simulink model "Simulation"  (R2023a)
settings: Solver=VariableStepAuto  StartTime=0.0  StopTime=100.0  RelTol=1e-3
settings Model: Creator=thoma  LastModifiedBy=cheva

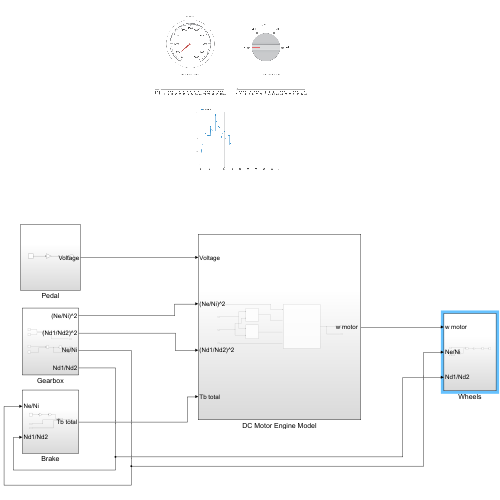
[thumbnail: Simulink's stored preview of the top-level diagram]
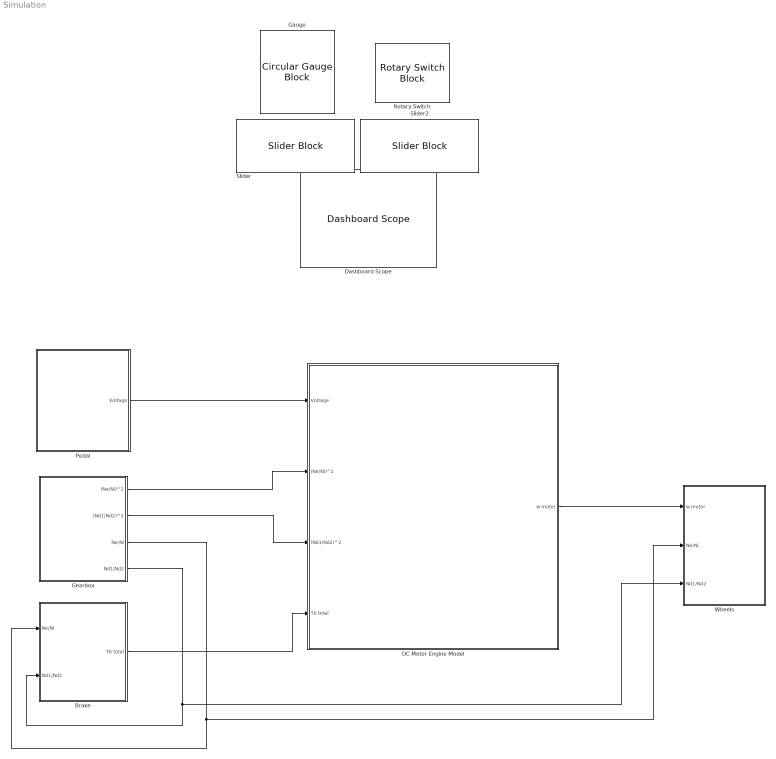
== system Simulation ==
  Brake : Subsystem
  DC Motor Engine Model : Subsystem
  Dashboard Scope : DashboardScope  Ymin=0  Ymax=10000
  Gauge : CircularGaugeBlock  ScaleMax=5000
  Gearbox : Subsystem
  Pedal : Subsystem
  Rotary Switch : RotarySwitchBlock
      settings: Values={{'1st', '2nd', '3rd', '4th'}, [3 2 1.5 1]}
  Slider : SliderBlock
  Slider2 : SliderBlock
  Wheels : Subsystem
  wires:
  Gearbox/4(Nd1/Nd2) -> Brake/2(Nd1/Nd2), Wheels/3(Nd1/Nd2)
  Gearbox/3(Ne/Ni) -> Brake/1(Ne/Ni), Wheels/2(Ne/Ni)
  Pedal/1(Voltage) -> DC Motor Engine Model/1(Voltage)
  Gearbox/1((Ne/Ni)^2) -> DC Motor Engine Model/2((Ne/Ni)^2)
  Gearbox/2((Nd1/Nd2)^2) -> DC Motor Engine Model/3((Nd1/Nd2)^2)
  Brake/1(Tb total) -> DC Motor Engine Model/4(Tb total)
  DC Motor Engine Model/1("w motor ") -> Wheels/1(w motor)

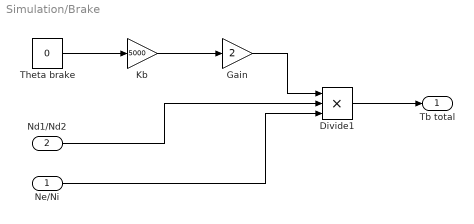
== system Simulation/Brake ==
  Ne/Ni : Inport
  Nd1/Nd2 : Inport  Port=2
  Divide1 : Product  Inputs=***
  Gain : Gain  Gain=2
  Kb : Gain  Gain=5000
  Theta brake : Constant  Value=0
  Tb total : Outport
  wires:
  Nd1/Nd2/1 -> Divide1/2
  Kb/1 -> Gain/1
  Ne/Ni/1 -> Divide1/3
  Theta brake/1 -> Kb/1
  Gain/1 -> Divide1/1
  Divide1/1 -> Tb total/1

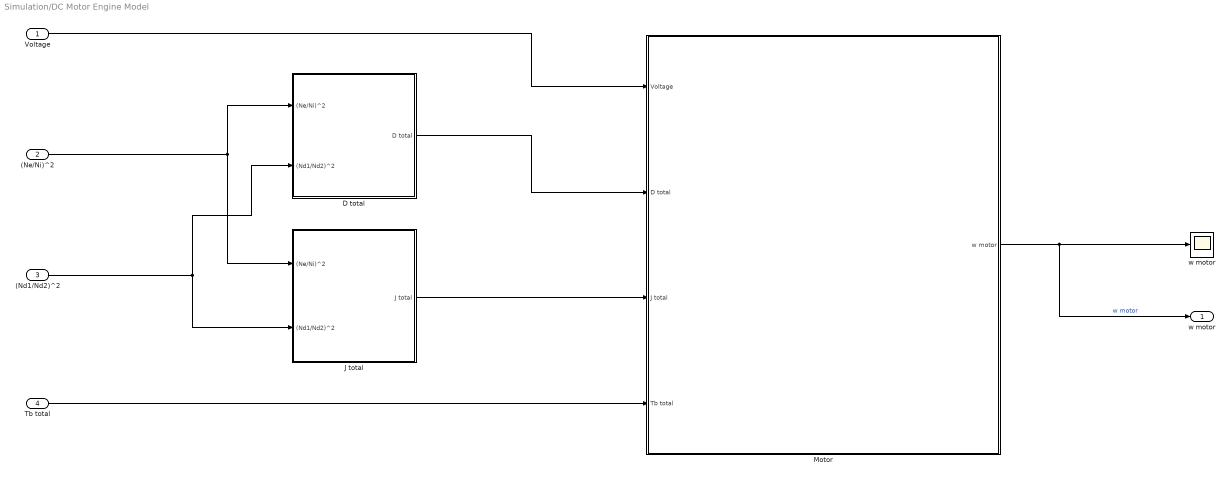
== system Simulation/DC Motor Engine Model ==
  Voltage : Inport
  (Ne/Ni)^2 : Inport  Port=2
  (Nd1/Nd2)^2 : Inport  Port=3
  Tb total : Inport  Port=4
  D total : Subsystem
  J total : Subsystem
  Motor : Subsystem
  w motor : Scope
  "w motor " : Outport
  wires:
  D total/1(D total) -> Motor/2(D total)
  J total/1(J total) -> Motor/3(J total)
  Motor/1(w motor) -> "w motor "/1, w motor/1  "w motor"
  Tb total/1 -> Motor/4(Tb total)
  Voltage/1 -> Motor/1(Voltage)
  (Nd1/Nd2)^2/1 -> D total/2((Nd1/Nd2)^2), J total/2((Nd1/Nd2)^2)
  (Ne/Ni)^2/1 -> J total/1((Ne/Ni)^2), D total/1((Ne/Ni)^2)

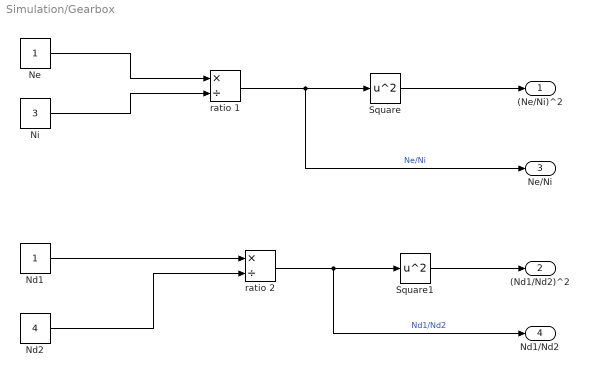
== system Simulation/Gearbox ==
  Nd1 : Constant
  Nd2 : Constant  Value=4
  Ne : Constant
  Ni : Constant  Value=3
  Square : Math  Operator=square
  Square1 : Math  Operator=square
  ratio 1 : Product  Inputs=*/
  ratio 2 : Product  Inputs=*/
  (Ne/Ni)^2 : Outport
  (Nd1/Nd2)^2 : Outport  Port=2
  Ne/Ni : Outport  Port=3
  Nd1/Nd2 : Outport  Port=4
  wires:
  Nd1/1 -> ratio 2/1
  ratio 1/1 -> Ne/Ni/1, Square/1  "Ne/Ni"
  Ni/1 -> ratio 1/2
  Nd2/1 -> ratio 2/2
  Ne/1 -> ratio 1/1
  ratio 2/1 -> Nd1/Nd2/1, Square1/1  "Nd1/Nd2"
  Square1/1 -> (Nd1/Nd2)^2/1
  Square/1 -> (Ne/Ni)^2/1

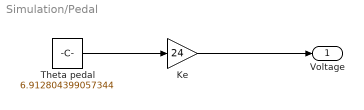
== system Simulation/Pedal ==
  Ke : Gain  Gain=24
  Theta pedal : Constant  Value=6.912804399057344
  Voltage : Outport
  wires:
  Ke/1 -> Voltage/1
  Theta pedal/1 -> Ke/1

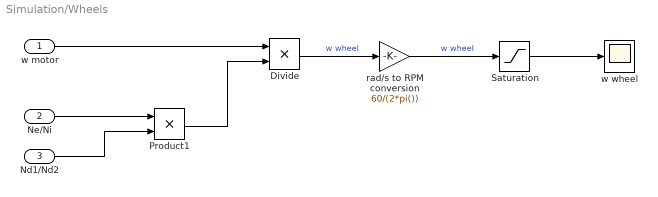
== system Simulation/Wheels ==
  w motor : Inport
  Ne/Ni : Inport  Port=2
  Nd1/Nd2 : Inport  Port=3
  Divide : Product  Inputs=**
  Product1 : Product
  Saturation : Saturate  UpperLimit=inf  LowerLimit=0
  rad/s to RPM conversion : Gain  Gain=60/(2*pi())
  w wheel : Scope
  wires:
  Divide/1 -> rad/s to RPM conversion/1  "w wheel"
  Product1/1 -> Divide/2
  rad/s to RPM conversion/1 -> Saturation/1  "w wheel"
  Nd1/Nd2/1 -> Product1/2
  Ne/Ni/1 -> Product1/1
  w motor/1 -> Divide/1
  Saturation/1 -> w wheel/1

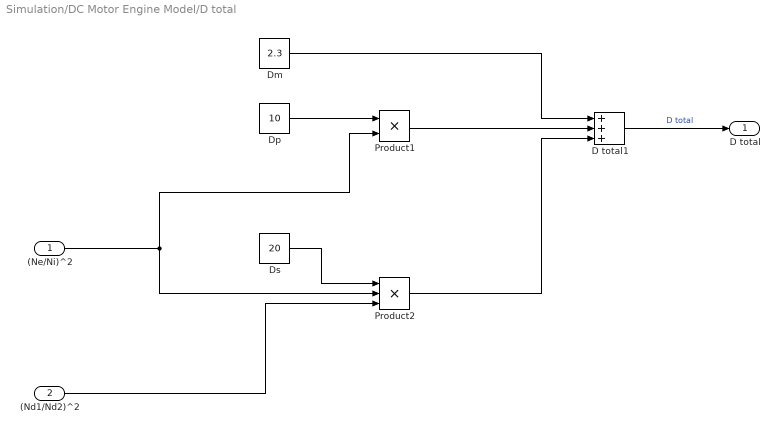
== system Simulation/DC Motor Engine Model/D total ==
  (Ne/Ni)^2 : Inport
  (Nd1/Nd2)^2 : Inport  Port=2
  D total1 : Sum  Inputs=+++
  Dm : Constant  Value=2.3
  Dp : Constant  Value=10
  Ds : Constant  Value=20
  Product1 : Product
  Product2 : Product  Inputs=3
  D total : Outport
  wires:
  Product1/1 -> D total1/2
  Dm/1 -> D total1/1
  Product2/1 -> D total1/3
  D total1/1 -> D total/1  "D total"
  Dp/1 -> Product1/1
  (Nd1/Nd2)^2/1 -> Product2/3
  (Ne/Ni)^2/1 -> Product1/2, Product2/2
  Ds/1 -> Product2/1

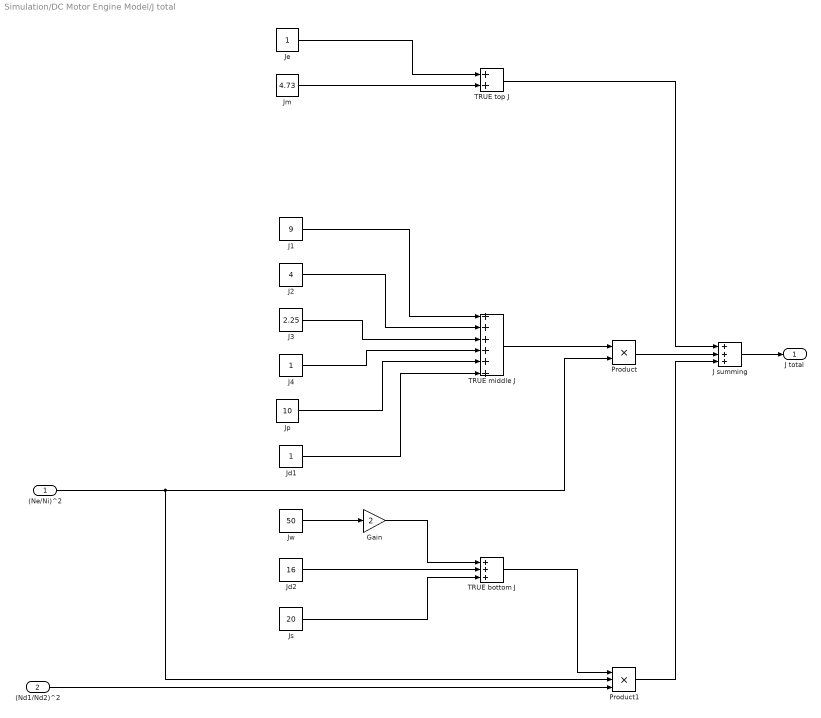
== system Simulation/DC Motor Engine Model/J total ==
  (Ne/Ni)^2 : Inport
  (Nd1/Nd2)^2 : Inport  Port=2
  Gain : Gain  Gain=2
  J summing : Sum  Inputs=+++
  J1 : Constant  Value=9
  J2 : Constant  Value=4
  J3 : Constant  Value=2.25
  J4 : Constant
  Jd1 : Constant
  Jd2 : Constant  Value=16
  Je : Constant
  Jm : Constant  Value=4.73
  Jp : Constant  Value=10
  Js : Constant  Value=20
  Jw : Constant  Value=50
  Product : Product
  Product1 : Product  Inputs=3
  TRUE bottom J : Sum  Inputs=+++
  TRUE middle J : Sum  Inputs=++++++
  TRUE top J : Sum
  J total : Outport
  wires:
  Product1/1 -> J summing/3
  TRUE top J/1 -> J summing/1
  Product/1 -> J summing/2
  J summing/1 -> J total/1
  Je/1 -> TRUE top J/1
  Jm/1 -> TRUE top J/2
  J2/1 -> TRUE middle J/2
  J3/1 -> TRUE middle J/3
  TRUE middle J/1 -> Product/1
  Jp/1 -> TRUE middle J/5
  Jd1/1 -> TRUE middle J/6
  J1/1 -> TRUE middle J/1
  J4/1 -> TRUE middle J/4
  (Ne/Ni)^2/1 -> Product1/2, Product/2
  Jw/1 -> Gain/1
  Js/1 -> TRUE bottom J/3
  (Nd1/Nd2)^2/1 -> Product1/3
  Jd2/1 -> TRUE bottom J/2
  TRUE bottom J/1 -> Product1/1
  Gain/1 -> TRUE bottom J/1

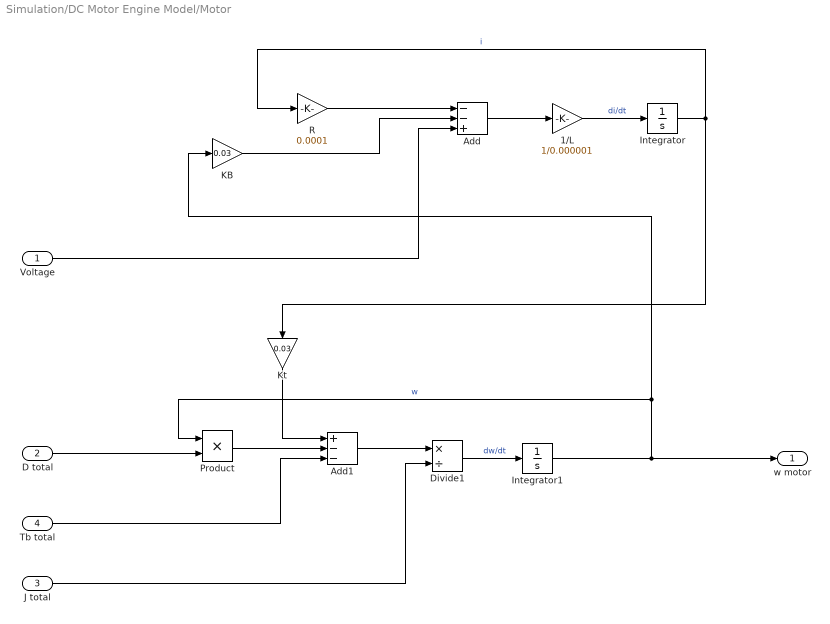
== system Simulation/DC Motor Engine Model/Motor ==
  Voltage : Inport
  D total : Inport  Port=2
  J total : Inport  Port=3
  Tb total : Inport  Port=4
  1/L : Gain  Gain=1/0.000001
  Add : Sum  Inputs=--+
  Add1 : Sum  Inputs=+--
  Divide1 : Product  Inputs=*/
  Integrator : Integrator
  Integrator1 : Integrator
  KB : Gain  Gain=0.03
  Kt : Gain  Gain=0.03
  Product : Product
  R : Gain  Gain=0.0001
  w motor : Outport
  wires:
  Kt/1 -> Add1/1
  Integrator/1 -> Kt/1, R/1  "i"
  KB/1 -> Add/2
  Product/1 -> Add1/2
  R/1 -> Add/1
  D total/1 -> Product/2
  Add/1 -> 1/L/1
  Divide1/1 -> Integrator1/1  "dw/dt"
  1/L/1 -> Integrator/1  "di/dt"
  Voltage/1 -> Add/3
  J total/1 -> Divide1/2
  Tb total/1 -> Add1/3
  Integrator1/1 -> KB/1, Product/1, w motor/1  "w"
  Add1/1 -> Divide1/1
